simulink model "Versuch_4_Reglergleichstrom"  (R2022b)
settings: Solver=VariableStepAuto  StartTime=0.0  StopTime=3  RelTol=1e-3
settings Model: Creator=janne  LastModifiedBy=janne

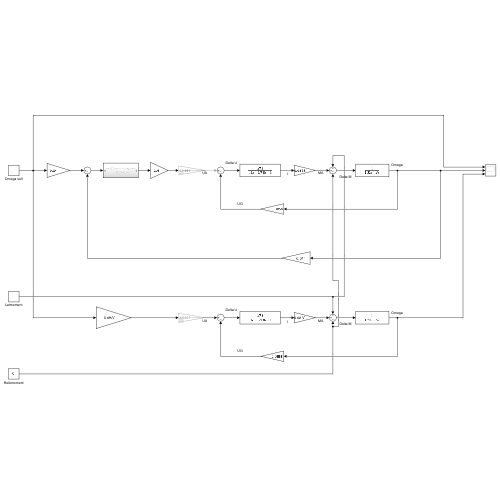
[thumbnail: Simulink's stored preview of the top-level diagram]
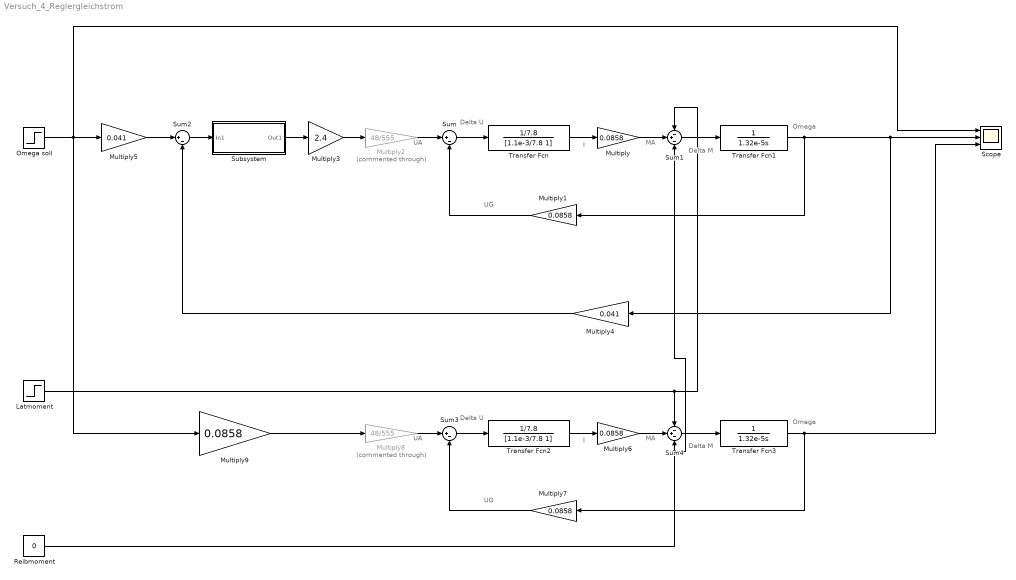
== system Versuch_4_Reglergleichstrom ==
  note: Omega
  note: UG
  note: Delta U
  note: I
  note: Delta M
  note: MA
  note: UA
  note: Omega
  note: UG
  note: Delta U
  note: MA
  note: I
  note: Delta M
  note: UA
  Latmoment : Step  After=0.052  SampleTime=0
  Multiply{,1,6..7,9} (5 alike) : Gain  Gain=0.0858
  Multiply2 : Gain  Commented=through  Gain=48/555
  Multiply3 : Gain  Gain=2.4
  Multiply4 : Gain  Gain=0.041
  Multiply5 : Gain  Gain=0.041
  Multiply8 : Gain  Commented=through  Gain=48/555
  Omega soll : Step  After=0  SampleTime=0
  Reibmoment : Constant  Value=0
  Scope : Scope  NumInputPorts=3
  Subsystem : Subsystem
  Sum : Sum  Inputs=|+-
  Sum1 : Sum  Inputs=-+-
  Sum2 : Sum  Inputs=|+-
  Sum3 : Sum  Inputs=|+-
  Sum4 : Sum  Inputs=-+-
  Transfer Fcn : TransferFcn  Numerator=1/7.8  Denominator=[1.1e-3/7.8 1]
  Transfer Fcn1 : TransferFcn  Denominator=[1.32e-5 0]
  Transfer Fcn2 : TransferFcn  Numerator=1/7.8  Denominator=[1.1e-3/7.8 1]
  Transfer Fcn3 : TransferFcn  Denominator=[1.32e-5 0]
  wires:
  Sum/1 -> Transfer Fcn/1
  Transfer Fcn/1 -> Multiply/1
  Multiply/1 -> Sum1/2
  Sum1/1 -> Transfer Fcn1/1
  Multiply1/1 -> Sum/2
  Multiply3/1 -> Multiply2/1
  Multiply2/1 -> Sum/1
  Multiply4/1 -> Sum2/2
  Multiply5/1 -> Sum2/1
  Transfer Fcn1/1 -> Multiply1/1, Scope/2, Multiply4/1
  Omega soll/1 -> Multiply9/1, Multiply5/1, Scope/1
  Multiply8/1 -> Sum3/1
  Transfer Fcn3/1 -> Multiply7/1, Scope/3
  Multiply7/1 -> Sum3/2
  Multiply6/1 -> Sum4/2
  Sum3/1 -> Transfer Fcn2/1
  Sum4/1 -> Transfer Fcn3/1
  Transfer Fcn2/1 -> Multiply6/1
  Latmoment/1 -> Sum1/1, Sum4/1
  Reibmoment/1 -> Sum1/3, Sum4/3
  Subsystem/1(Out1) -> Multiply3/1
  Sum2/1 -> Subsystem/1(In1)
  Multiply9/1 -> Multiply8/1

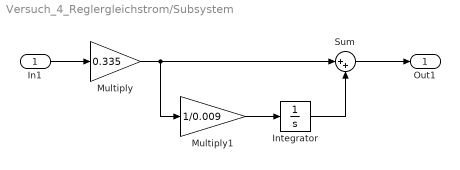
== system Versuch_4_Reglergleichstrom/Subsystem ==
  In1 : Inport
  Integrator : Integrator
  Multiply : Gain  Gain=0.335
  Multiply1 : Gain  Gain=1/0.009
  Sum : Sum  Inputs=|++
  Out1 : Outport
  wires:
  Multiply1/1 -> Integrator/1
  Multiply/1 -> Multiply1/1, Sum/1
  Integrator/1 -> Sum/2
  Sum/1 -> Out1/1
  In1/1 -> Multiply/1
